simulink model "freedm_vs2"  (Simulink 9.2)
settings: Solver=ode45  StartTime=0.0  StopTime=Tmax  RelTol=1e-3  EnableMultiTasking=on
values from neighbouring files (symbols this model uses):
  Bmax = 50    [para.m]
  d2 = 0    [para.m]
  grm0 = 0    [para.m]
  maxm = 2    [para.m]
  r1 = 3    [para.m]
  r2 = 3    [para.m]
  thresh = 5    [para.m]
settings Model: Creator=Luan Nguyen  LastModifiedBy=LuanNguyen
settings OptimizationCC: ExpressionDepthLimit=2147483647
settings DebuggingCC: MultiTaskDSMMsg=warning  MultiTaskCondExecSysMsg=none  FcnCallInpInsideContextMsg=error
settings GRTTargetCC: CombineOutputUpdateFcns=on  GRTInterface=off
settings ConfigComp: CovSFcnEnable=off

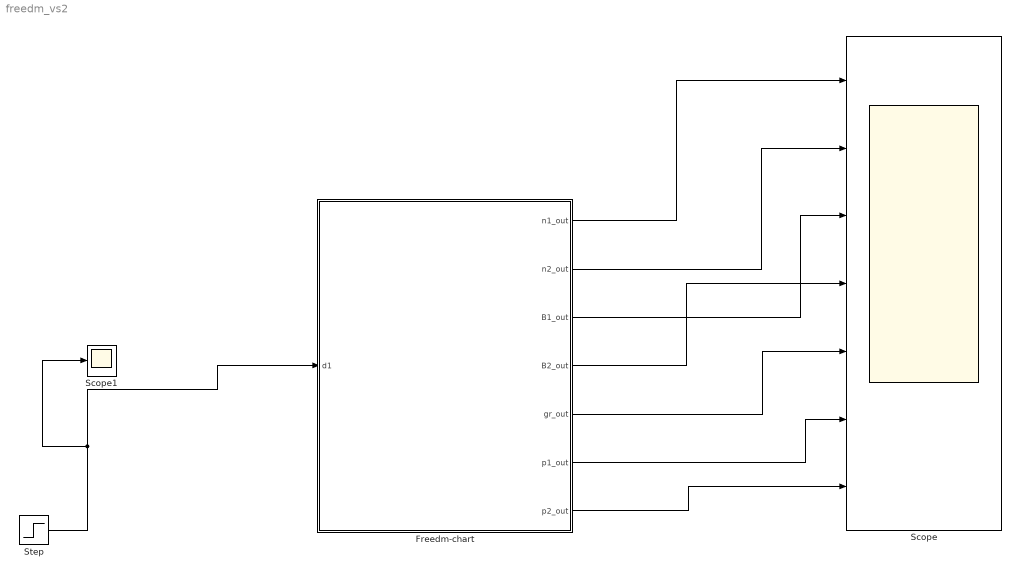
== system freedm_vs2 ==
  Freedm-chart : Stateflow chart  TreatAsAtomicUnit=on
  Scope : Scope  NumInputPorts=7
  Scope1 : Scope
  Step : Step  Time=10  Before=10  After=0  SampleTime=0
  wires:
  Freedm-chart/1(n1_out) -> Scope/1
  Freedm-chart/2(n2_out) -> Scope/2
  Freedm-chart/3(B1_out) -> Scope/3
  Freedm-chart/4(B2_out) -> Scope/4
  Freedm-chart/5(gr_out) -> Scope/5
  Freedm-chart/6(p1_out) -> Scope/6
  Freedm-chart/7(p2_out) -> Scope/7
  Step/1 -> Freedm-chart/1(d1), Scope1/1

== stateflow chart Freedm-chart ==
  settings: updateMethod=CONTINUOUS
  state Migrate [parallel]
    settings: executionOrder=3
    state Migrate2 [parallel]
      settings: executionOrder=2
      state Mode21
      state Mode22
      (default) -> Mode22
      Mode21 -> Mode22 : [d2 - (r2+p2) < thresh || d1 - (r1+p1) >= 0]
          | {m = 0;}
      Mode22 -> Mode21 : [d2 - (r2+p2) >= thresh && d1 - (r1+p1) < 0]
          | {m = maxm; }
    state Migrate1 [parallel]
      settings: executionOrder=1
      state Mode11
      state Mode12
      (default) -> Mode12
      Mode11 -> Mode12 : [d1 - (r1+p1) < thresh || d2 - (r2+p2) >= 0]
          | {m = 0;}
      Mode12 -> Mode11 : [d1 - (r1+p1) >= thresh && d2 - (r2+p2) < 0]
          | {m = -maxm; }
  state Battery_controller [parallel]
    settings: executionOrder=4
    state Bat1 [parallel]
      settings: executionOrder=1
      state To_grid1
      state To_bat1
      (default) -> To_grid1
      To_bat1 -> To_grid1 : [!(d1 - (r1+p1) <= 0 && B1 < Bmax) && !(d1 - (r1+p1) > 0 && B1 > 0)]
          | {b1 = 0; gr = gr - (d1 - (r1+p1)); grm = grm + m;}
      To_grid1 -> To_bat1 : [(d1 - (r1+p1) <= 0 && B1 < Bmax) || (d1 - (r1+p1)> 0 && B1 > 0)]
          | {b1 = -(d1 - (r1+p1)); bm1 = bm1+m;}
    state Bat2 [parallel]
      settings: executionOrder=2
      state To_bat2
      state To_grid2
      (default) -> To_grid2
      To_bat2 -> To_grid2 : [(d2 - (r2+p2) > 0 || B2 >= Bmax) && (d2 - (r2+p2) <= 0 || B2 <= 0)]
          | {b2 = 0; gr = gr - (d2 - (r2+p2)); grm = grm - m;}
      To_grid2 -> To_bat2 : [(d2 - (r2+p2) <= 0 && B2 < Bmax)|| (d2 - (r2+p2) > 0 && B2 > 0)]
          | {b2 = -(d2 - (r2+p2)); bm2 = bm2-m;}
  state plant1 [parallel]
    settings: executionOrder=1
    state Plan11
      du:
      p1_dot = -m; B1_dot = b1; b1_dot = bm1; gr_dot = grm;
      t_dot = 1;
      gr_out = gr;
      B1_out = B1;
      p1_out = p1;
      n1_out = d1 - (r1+p1);
    state Plan12
      du:
      p1_dot = -m; B1_dot = b1; b1_dot = bm1; gr_dot = grm;
      t_dot = 1;
      gr_out = gr;
      B1_out = B1;
      p1_out = p1;
      n1_out = d1 - (r1+p1);
    (default) -> Plan11 : {p1 = 0; b1 = 0; m = 0; B1 = Bmax;gr = 0; t = 0; p2 = 0; b2 = 0; B2 = 0.8*Bmax; grm = grm0; bm1 = 0; bm2 = 0;}
    Plan11 -> Plan12 : [B1 < 0 ||  B1 > Bmax]
        | {b1 =0; bm1 = 0}
    Plan12 -> Plan11 : [!(B1 < 0 ||  B1 > Bmax)]
  state plant2 [parallel]
    settings: executionOrder=2
    state Plan22
      du:
      p2_dot = m; B2_dot = b2; b2_dot = bm2;
      B2_out = B2;
      p2_out = p2;
      n2_out = d2 - (r2+p2);
    state Plan21
      du:
      p2_dot = m; B2_dot = b2; b2_dot = bm2;
      B2_out = B2;
      p2_out = p2;
      n2_out = d2 - (r2+p2);
    Plan21 -> Plan22 : [B2 < 0 ||  B2 > Bmax]
        | {b2 =0; bm2 = 0}
    (default) -> Plan21
    Plan22 -> Plan21 : [!(B2 < 0 ||  B2 > Bmax)]
  data: t local double; p1 local double; p2 local double; n1_out output double; Bmax parameter double; B1 local double; B2 local double; b1 local double; b2 local double; n2_out output double; grm local double; d2 parameter double; r1 parameter double; r2 parameter double; maxm parameter double; thresh parameter double; B1_out output double; B2_out output double; bm1 local double; bm2 local double; gr local double; gr_out output double; m local double; grm0 parameter double; p1_out output double; p2_out output double; d1 input double
  data t settings: updateMethod=SF_CONTINUOUS_TIME_DATA
  data p1 settings: updateMethod=SF_CONTINUOUS_TIME_DATA
  data p2 settings: updateMethod=SF_CONTINUOUS_TIME_DATA
  data B1 settings: updateMethod=SF_CONTINUOUS_TIME_DATA
  data B2 settings: updateMethod=SF_CONTINUOUS_TIME_DATA
  data b1 settings: updateMethod=SF_CONTINUOUS_TIME_DATA
  data b2 settings: updateMethod=SF_CONTINUOUS_TIME_DATA
  data gr settings: updateMethod=SF_CONTINUOUS_TIME_DATA
